simulink model "Model_XSAO2"  (Simulink 7.0)
settings: Solver=ode45  StartTime="    0.0167"  StopTime=7.6  MaxStep=0.001  RelTol=1e-3  AbsTol=1e-3
values from neighbouring files (symbols this model uses):
  Ad = [Adop(1); A]    [sa_ta_optim.m]    (also in sur_opt.m)
  DOd = [O2dop(1); DOd; O2dop(2)]    [sa_ta_optim.m]    (also in sur_opt.m)
  F = ec1807kf(ndx,6)    [sa_ta_optim.m]    (also in sur_opt.m)
  K1 = par(3)    [error_sa_ta.m]    (also in sa_ta_optim.m = par1(3); sur_opt.m = xm(3))
  Ks = par(2)    [error_sa_ta.m]    (also in sa_ta_optim.m = par1(2); sur_opt.m = xm(2))
  Mmax = par(1)    [error_sa_ta.m]    (also in sa_ta_optim.m = par1(1); sur_opt.m = xm(1))
  N = 40    [sur_opt.m]
  Sd = ec1807kf(ndx,2)    [sa_ta_optim.m]    (also in sur_opt.m = interp1(t, Sd, Tt1))
  V = ec1807k(ndx,6)    [sa_ta_optim.m]    (also in sur_opt.m)
  Xd = ec1807kf(ndx,3)    [sa_ta_optim.m]    (also in sur_opt.m = interp1(t, Xd, Tt1))
undefined symbols (not defined in the file or in its folder): DOo, K2, K3, Kla, So
settings Model: Creator=Olympia Roeva  LastModifiedBy=Olympia Roeva  ExtModeTrigMode=oneshot  ExtModeArmWhenConnect=off
settings DataIOCC: LimitDataPoints=off  SaveOutput=off  SaveTime=off
settings OptimizationCC: BlockReduction=off  BooleanDataType=off
settings DebuggingCC: SaveWithParameterizedLinksMsg=none  SignalResolutionControl=TryResolveAllWithWarning  SolverPrmCheckMsg=none  MultiTaskDSMMsg=warning  MultiTaskCondExecSysMsg=none  StrictBusMsg=None
settings HardwareCC: TargetUnknown=on
settings RTWCC: IncludeERTFirstTime=on

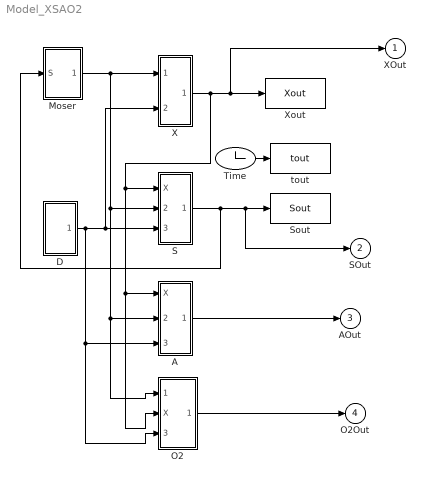
== system Model_XSAO2 ==
  A : Subsystem
  D : Subsystem
  Moser : Subsystem
  O2 : Subsystem
  S : Subsystem
  Sout : ToWorkspace  VariableName=Sout  SampleTime=-1  SaveFormat=Array
  Time : Clock
      settings: Decimation=10
  X : Subsystem
  Xout : ToWorkspace  VariableName=Xout  SampleTime=-1  SaveFormat=Array
  tout : ToWorkspace  VariableName=tout  SampleTime=-1  SaveFormat=Array
  XOut : Outport
  SOut : Outport  Port=2
  AOut : Outport  Port=3
  O2Out : Outport  Port=4
  wires:
  X/1(XOut) -> Xout/1, XOut/1, S/1(X), A/1(X), O2/2(X)
  S/1(Sout) -> Sout/1, SOut/1, Moser/1(S)
  Time/1 -> tout/1
  Moser/1(mu) -> X/1(mu), S/2(mu), A/2(mu), O2/1(mu)
  D/1(out_1) -> S/3(F/V), X/2(F/V), A/3(F/V), O2/3(F/V)
  O2/1(DOout) -> O2Out/1
  A/1(Aout) -> AOut/1

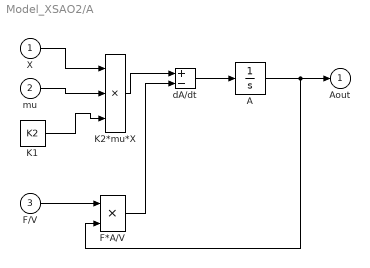
== system Model_XSAO2/A ==
  X : Inport
  mu : Inport  Port=2
  F/V : Inport  Port=3
  A : Integrator  InitialCondition=Ad(1)
  F*A/V : Product  SaturateOnIntegerOverflow=on  RndMeth=Zero  InputSameDT=on
  K1 : Constant  Value=K2
  K2*mu*X : Product  Inputs=3  SaturateOnIntegerOverflow=on  RndMeth=Zero  InputSameDT=on
  dA/dt : Sum  Inputs=+-  SaturateOnIntegerOverflow=on  InputSameDT=on
  Aout : Outport
  wires:
  A/1 -> Aout/1, F*A/V/2
  dA/dt/1 -> A/1
  K2*mu*X/1 -> dA/dt/1
  X/1 -> K2*mu*X/1
  mu/1 -> K2*mu*X/2
  F/V/1 -> F*A/V/1
  F*A/V/1 -> dA/dt/2
  K1/1 -> K2*mu*X/3

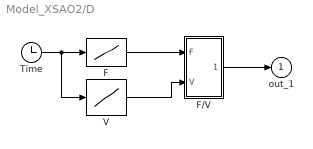
== system Model_XSAO2/D ==
  F : Lookup  InputValues=t  Table=F  SaturateOnIntegerOverflow=on
  F/V : Subsystem
      mask Type: /
      mask Description: Division of two scalars. y=u[1]/u[2]
      mask Help: Division of two scalars: y=u[1]/u[2]
      mask Display: disp('/')
  Time : Clock
      settings: Decimation=10
  V : Lookup  InputValues=t  Table=V  SaturateOnIntegerOverflow=on
  out_1 : Outport
  wires:
  F/V/1(out_1) -> out_1/1
  F/1 -> F/V/1(F)
  V/1 -> F/V/2(V)
  Time/1 -> F/1, V/1

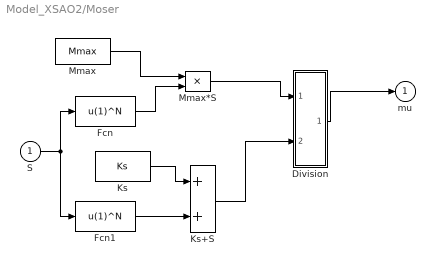
== system Model_XSAO2/Moser ==
  S : Inport
  Division : Subsystem
      mask Type: /
      mask Description: Division of two scalars. y=u[1]/u[2]
      mask Help: Division of two scalars: y=u[1]/u[2]
      mask Display: disp('/')
  Fcn : Fcn  Expr=u(1)^N
  Fcn1 : Fcn  Expr=u(1)^N
  Ks : Constant  Value=Ks
  Ks+S : Sum  SaturateOnIntegerOverflow=on  InputSameDT=on
  Mmax : Constant  Value=Mmax
  Mmax*S : Product  SaturateOnIntegerOverflow=on  RndMeth=Zero  InputSameDT=on
  mu : Outport
  wires:
  Division/1(out_1) -> mu/1
  Mmax/1 -> Mmax*S/1
  Mmax*S/1 -> Division/1(Mmax*S)
  Ks+S/1 -> Division/2(Ks+S)
  Ks/1 -> Ks+S/1
  S/1 -> Fcn/1, Fcn1/1
  Fcn/1 -> Mmax*S/2
  Fcn1/1 -> Ks+S/2

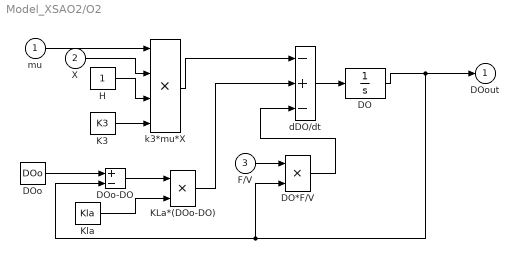
== system Model_XSAO2/O2 ==
  mu : Inport
  X : Inport  Port=2
  F/V : Inport  Port=3
  DO : Integrator  InitialCondition=DOd(1)  UpperSaturationLimit=1000  LowerSaturationLimit=0
  DO*F/V : Product  SaturateOnIntegerOverflow=on  RndMeth=Zero  InputSameDT=on
  DOo : Constant  Value=DOo
  DOo-DO : Sum  Inputs=+-  SaturateOnIntegerOverflow=on  InputSameDT=on
  H : Constant
  K3 : Constant  Value=K3
  KLa*(DOo-DO) : Product  SaturateOnIntegerOverflow=on  RndMeth=Zero  InputSameDT=on
  Kla : Constant  Value=Kla
  dDO/dt : Sum  Inputs=-+-  SaturateOnIntegerOverflow=on  InputSameDT=on
  k3*mu*X : Product  Inputs=4  SaturateOnIntegerOverflow=on  RndMeth=Zero  InputSameDT=on
  DOout : Outport
  wires:
  DO/1 -> DOout/1, DOo-DO/2, DO*F/V/2
  dDO/dt/1 -> DO/1
  k3*mu*X/1 -> dDO/dt/1
  mu/1 -> k3*mu*X/1
  X/1 -> k3*mu*X/2
  H/1 -> k3*mu*X/3
  K3/1 -> k3*mu*X/4
  KLa*(DOo-DO)/1 -> dDO/dt/2
  DOo-DO/1 -> KLa*(DOo-DO)/1
  DOo/1 -> DOo-DO/1
  Kla/1 -> KLa*(DOo-DO)/2
  F/V/1 -> DO*F/V/1
  DO*F/V/1 -> dDO/dt/3

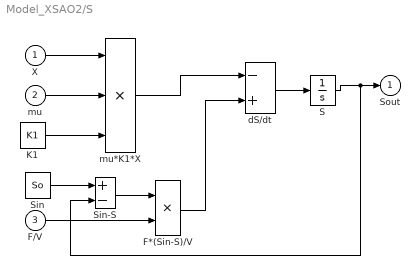
== system Model_XSAO2/S ==
  X : Inport
  mu : Inport  Port=2
  F/V : Inport  Port=3
  F*(Sin-S)/V : Product  SaturateOnIntegerOverflow=on  RndMeth=Zero  InputSameDT=on
  K1 : Constant  Value=K1
  S : Integrator  InitialCondition=Sd(1)  UpperSaturationLimit=1000  LowerSaturationLimit=0
  Sin : Constant  Value=So
  Sin-S : Sum  Inputs=+-  SaturateOnIntegerOverflow=on  InputSameDT=on
  dS/dt : Sum  Inputs=-+  SaturateOnIntegerOverflow=on  InputSameDT=on
  mu*K1*X : Product  Inputs=3  SaturateOnIntegerOverflow=on  RndMeth=Zero  InputSameDT=on
  Sout : Outport
  wires:
  S/1 -> Sout/1, Sin-S/2
  Sin-S/1 -> F*(Sin-S)/V/1
  Sin/1 -> Sin-S/1
  X/1 -> mu*K1*X/1
  F/V/1 -> F*(Sin-S)/V/2
  mu*K1*X/1 -> dS/dt/1
  F*(Sin-S)/V/1 -> dS/dt/2
  dS/dt/1 -> S/1
  mu/1 -> mu*K1*X/2
  K1/1 -> mu*K1*X/3

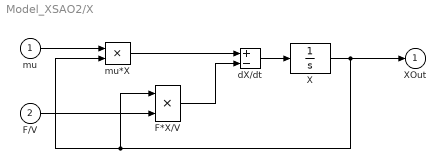
== system Model_XSAO2/X ==
  mu : Inport
  F/V : Inport  Port=2
  F*X/V : Product  SaturateOnIntegerOverflow=on  RndMeth=Zero  InputSameDT=on
  X : Integrator  InitialCondition=Xd(1)  UpperSaturationLimit=1000  LowerSaturationLimit=0
  dX/dt : Sum  Inputs=+-  SaturateOnIntegerOverflow=on  InputSameDT=on
  mu*X : Product  SaturateOnIntegerOverflow=on  RndMeth=Zero  InputSameDT=on
  XOut : Outport
  wires:
  F*X/V/1 -> dX/dt/2
  dX/dt/1 -> X/1
  mu*X/1 -> dX/dt/1
  mu/1 -> mu*X/1
  X/1 -> XOut/1, mu*X/2, F*X/V/1
  F/V/1 -> F*X/V/2

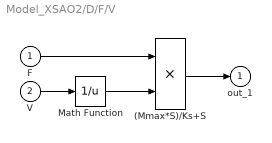
== system Model_XSAO2/D/F/V ==
  F : Inport
  V : Inport  Port=2
  (Mmax*S)/Ks+S : Product  SaturateOnIntegerOverflow=on  RndMeth=Zero  InputSameDT=on
  Math Function : Math  Operator=reciprocal  SaturateOnIntegerOverflow=on
  out_1 : Outport
  wires:
  F/1 -> (Mmax*S)/Ks+S/1
  V/1 -> Math Function/1
  Math Function/1 -> (Mmax*S)/Ks+S/2
  (Mmax*S)/Ks+S/1 -> out_1/1

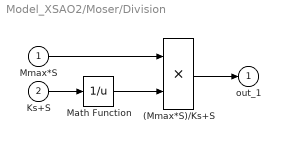
== system Model_XSAO2/Moser/Division ==
  Mmax*S : Inport
  Ks+S : Inport  Port=2
  (Mmax*S)/Ks+S : Product  SaturateOnIntegerOverflow=on  RndMeth=Zero  InputSameDT=on
  Math Function : Math  Operator=reciprocal  SaturateOnIntegerOverflow=on
  out_1 : Outport
  wires:
  Mmax*S/1 -> (Mmax*S)/Ks+S/1
  Ks+S/1 -> Math Function/1
  Math Function/1 -> (Mmax*S)/Ks+S/2
  (Mmax*S)/Ks+S/1 -> out_1/1
